simulink model "CM4_IMU_Test"  (R2020b)
settings: Solver=FixedStepAuto  StartTime=0.0  StopTime=60  FixedStep=0.01  RelTol=1e-3  EnableMultiTasking=on
libraries: simulink x6, raspberrypiCommlib x2
settings Model: Creator=cbeal  LastModifiedBy=cbeal
settings SolverCC: PositivePriorityOrder=on
settings OptimizationCC: EnhancedBackFolding=on  PassReuseOutputArgsAs=Individual arguments  ZeroExternalMemoryAtStartup=off  ZeroInternalMemoryAtStartup=off  MaxStackSize=64  OptimizeBlockOrder=speed  DifferentSizesBufferReuse=on  OptimizationCustomize=off  EfficientTunableParamExpr=on
settings DebuggingCC: ParameterTunabilityLossMsg=error
settings HardwareCC: ProdBitPerPointer=32  ProdBitPerSizeT=32  ProdBitPerPtrDiffT=32  ProdLargestAtomicInteger=Long  ProdLargestAtomicFloat=Double  ProdWordSize=32  ProdLongLongMode=on  ProdHWDeviceType=ARM Compatible->ARM Cortex
settings RTWCC: Description=Embedded Coder  SystemTargetFile=ert.tlc  HardwareBoard=Raspberry Pi  TLCOptions="-aInlineSetEventsForThisBaseRateFcn=TLC_FALSE -aSuppressMultiTaskScheduler=TLC_FALSE  -aRateBasedStepFcn=0"  TemplateMakefile=ert_default_tmf  Toolchain=GNU GCC Raspberry Pi  BuildConfiguration=Faster Runs
settings CodeAppCC: ForceParamTrailComments=on  IgnoreCustomStorageClasses=off  OperatorAnnotations=on  SimulinkDataObjDesc=on  SFDataObjDesc=on  InsertBlockDesc=on
settings ERTTargetCC: MatFileLogging=on  SupportVariableSizeSignals=on  ExtModeTransport=2  ExtModeMexFile=ext_xcp  ExtModeIntrfLevel=Level2 - Open

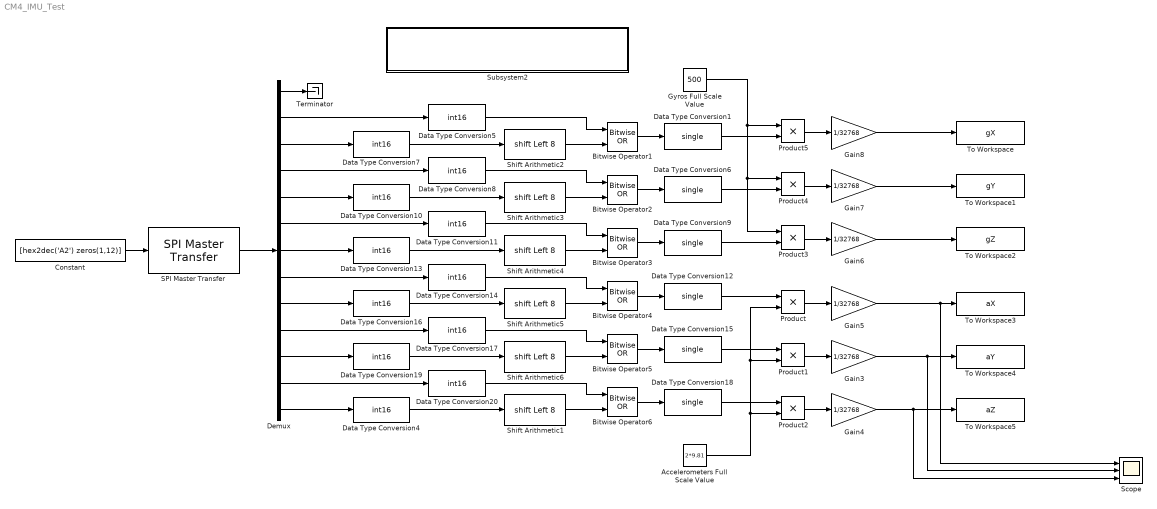
== system CM4_IMU_Test ==
  Accelerometers Full Scale Value : Constant  Value=2*9.81
  Bitwise Operator{1..6} (6 alike) : simulink/Logic and Bit Operations/Bitwise Operator  logicop=OR  UseBitMask=off  NumInputPorts=2  BitMask=bin2dec('11011001')  BitMaskRealWorld=Stored Integer
  Constant : Constant  Value=[hex2dec('A2') zeros(1,12)]  OutDataTypeStr=uint8
  Data Type Conversion{1,6,9,12,15,18} (6 alike) : DataTypeConversion  OutDataTypeStr=single
  Data Type Conversion{4..5,7..8,10..11,13..14,16..17,19..20} (12 alike) : DataTypeConversion  OutDataTypeStr=int16  ConvertRealWorld=Stored Integer (SI)
  Demux : Demux  Outputs=13
  Gain{3..8} (6 alike) : Gain  Gain=1/32768
  Gyros Full Scale Value : Constant  Value=500
  Product{,1..5} (6 alike) : Product
  SPI Master Transfer : raspberrypiCommlib/SPI Master Transfer  BoardProperty=Pi 4 Model B  SPIModule=SPI1  Mode=Master  BusSpeed=1000000  Pin=uint32(0)  FirstBitToTransfer=Most significant bit (MSB)  ClockMode=0  BlockFunction=Transfer  RegisterAddress=0  OutputDataType=int8  OutputDataLength=1  SSPin=CS2
      settings: SourceProductBaseCode=RASPPI
  Scope : Scope  NumInputPorts=3
  Shift Arithmetic{1..6} (6 alike) : ArithShift  BitShiftNumber=8  BitShiftDirection=Left
  Subsystem2 : Subsystem
      mask Display:
      | scl=1/4;
      | patch(scl*[0,52,90,54],scl*[16,55,146,146],[16/255,118/255,188/255],'bottom-left');
      | patch(scl*[0,27,82,77,68],scl*[16,0,42,62,69],[46/255,49/255,146/255],'bottom-left');
      | patch(scl*[89,125,90,68],scl*[16,16,146,91],[0,0,0],'bottom-left');
      | disp('Run Once at Startup');
  Terminator : Terminator
  To Workspace : ToWorkspace  VariableName=gX  SampleTime=-1
      settings: Save2DSignal=2-D array (concatenate along first dimension)
  To Workspace1 : ToWorkspace  VariableName=gY  SampleTime=-1
      settings: Save2DSignal=2-D array (concatenate along first dimension)
  To Workspace2 : ToWorkspace  VariableName=gZ  SampleTime=-1
      settings: Save2DSignal=2-D array (concatenate along first dimension)
  To Workspace3 : ToWorkspace  VariableName=aX  SampleTime=-1
      settings: Save2DSignal=2-D array (concatenate along first dimension)
  To Workspace4 : ToWorkspace  VariableName=aY  SampleTime=-1
      settings: Save2DSignal=2-D array (concatenate along first dimension)
  To Workspace5 : ToWorkspace  VariableName=aZ  SampleTime=-1
      settings: Save2DSignal=2-D array (concatenate along first dimension)
  wires:
  Gain5/1 -> Scope/1, To Workspace3/1
  Data Type Conversion16/1 -> Shift Arithmetic5/1
  Data Type Conversion19/1 -> Shift Arithmetic6/1
  Gain6/1 -> To Workspace2/1
  Gain7/1 -> To Workspace1/1
  Product3/1 -> Gain6/1
  Product5/1 -> Gain8/1
  Gain4/1 -> Scope/3, To Workspace5/1
  Gain8/1 -> To Workspace/1
  Product4/1 -> Gain7/1
  Gyros Full Scale Value/1 -> Product5/1, Product4/1, Product3/1
  Product2/1 -> Gain4/1
  Bitwise Operator6/1 -> Data Type Conversion18/1
  Data Type Conversion12/1 -> Product/1
  Accelerometers Full Scale Value/1 -> Product2/2, Product1/2, Product/2
  Bitwise Operator4/1 -> Data Type Conversion12/1
  Data Type Conversion6/1 -> Product4/2
  Bitwise Operator1/1 -> Data Type Conversion1/1
  Data Type Conversion9/1 -> Product3/2
  Product1/1 -> Gain3/1
  Data Type Conversion13/1 -> Shift Arithmetic4/1
  Data Type Conversion18/1 -> Product2/1
  Data Type Conversion15/1 -> Product1/1
  Data Type Conversion10/1 -> Shift Arithmetic3/1
  Data Type Conversion1/1 -> Product5/2
  Bitwise Operator3/1 -> Data Type Conversion9/1
  Product/1 -> Gain5/1
  Data Type Conversion4/1 -> Shift Arithmetic1/1
  Bitwise Operator2/1 -> Data Type Conversion6/1
  Data Type Conversion7/1 -> Shift Arithmetic2/1
  Bitwise Operator5/1 -> Data Type Conversion15/1
  Gain3/1 -> Scope/2, To Workspace4/1
  Constant/1 -> SPI Master Transfer/1
  Demux/1 -> Terminator/1
  SPI Master Transfer/1 -> Demux/1
  Shift Arithmetic2/1 -> Bitwise Operator1/2
  Shift Arithmetic3/1 -> Bitwise Operator2/2
  Shift Arithmetic4/1 -> Bitwise Operator3/2
  Shift Arithmetic5/1 -> Bitwise Operator4/2
  Shift Arithmetic6/1 -> Bitwise Operator5/2
  Shift Arithmetic1/1 -> Bitwise Operator6/2
  Data Type Conversion20/1 -> Bitwise Operator6/1
  Data Type Conversion17/1 -> Bitwise Operator5/1
  Data Type Conversion5/1 -> Bitwise Operator1/1
  Data Type Conversion8/1 -> Bitwise Operator2/1
  Data Type Conversion11/1 -> Bitwise Operator3/1
  Data Type Conversion14/1 -> Bitwise Operator4/1
  Demux/2 -> Data Type Conversion5/1
  Demux/3 -> Data Type Conversion7/1
  Demux/4 -> Data Type Conversion8/1
  Demux/5 -> Data Type Conversion10/1
  Demux/6 -> Data Type Conversion11/1
  Demux/7 -> Data Type Conversion13/1
  Demux/8 -> Data Type Conversion14/1
  Demux/9 -> Data Type Conversion16/1
  Demux/10 -> Data Type Conversion17/1
  Demux/11 -> Data Type Conversion19/1
  Demux/12 -> Data Type Conversion20/1
  Demux/13 -> Data Type Conversion4/1

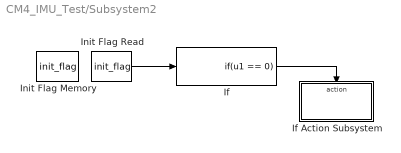
== system CM4_IMU_Test/Subsystem2 ==
  If : If  IfExpression=u1 == 0  ShowElse=off
  If Action Subsystem : Subsystem  TreatAsAtomicUnit=on
  Init Flag Memory : DataStoreMemory  DataStoreName=init_flag  ReadBeforeWriteMsg=warning  WriteAfterWriteMsg=warning  WriteAfterReadMsg=warning  ShowAdditionalParam=off  OutDataTypeStr=uint32
  Init Flag Read : DataStoreRead  DataStoreName=init_flag
  wires:
  Init Flag Read/1 -> If/1
  If/1 -> If Action Subsystem/Action

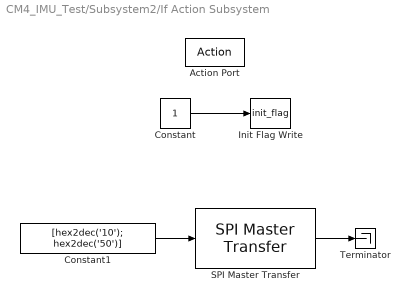
== system CM4_IMU_Test/Subsystem2/If Action Subsystem ==
  Action Port : ActionPort  ActionPortLabel=if(u1 == 0)
  Constant : Constant  OutDataTypeStr=uint32
  Constant1 : Constant  Value=[hex2dec('10'); hex2dec('50')]  OutDataTypeStr=uint8
  Init Flag Write : DataStoreWrite  DataStoreName=init_flag
  SPI Master Transfer : raspberrypiCommlib/SPI Master Transfer  BoardProperty=Pi 4 Model B  SPIModule=SPI1  Mode=Master  BusSpeed=1000000  Pin=uint32(0)  FirstBitToTransfer=Most significant bit (MSB)  ClockMode=0  BlockFunction=Transfer  RegisterAddress=0  OutputDataType=int8  OutputDataLength=1  SSPin=CS2
      settings: SourceProductBaseCode=RASPPI
  Terminator : Terminator
  wires:
  Constant/1 -> Init Flag Write/1
  Constant1/1 -> SPI Master Transfer/1
  SPI Master Transfer/1 -> Terminator/1
